simulink model "Carousel_SImulator"  (R2025a)
settings: Solver=VariableStepAuto  StartTime=0.0  StopTime=10.0  RelTol=1e-3
values from neighbouring files (symbols this model uses):
  initial_guess = homeConfiguration(robot)    [ik_solver_setup.m]
undefined symbols (not defined in the file or in its folder): exprnd, m, n, System
settings Model: Creator=samadhan  LastModifiedBy=samadhan

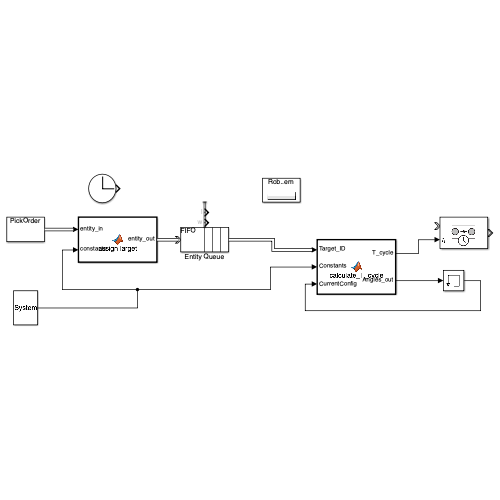
[thumbnail: Simulink's stored preview of the top-level diagram]
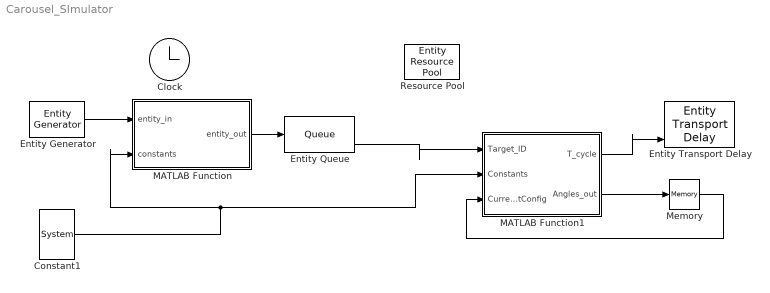
== system Carousel_SImulator ==
  Clock : Clock
  Constant1 : Constant  Value=System
  Entity Transport Delay : EntityTransportDelay  InputPortMessageModes=m,n  OutputPortMessageModes=m
  Entity Generator : EntityGenerator  OutputPortMessageModes=m  Period=eval('exprnd(10)')  IntergenerationTimeAction=exprnd(10)  AttributeName=Target_Bin_ID  EntityType=Structured  EntityTypeName=PickOrder  EntityPriority=1
  Entity Queue : Queue  InputPortMessageModes=m  OutputPortMessageModes=n,n,m  Capacity=inf  AverageWait=on  AverageQueueLength=on
      settings: OutputPortMap=o2,o3,o5
  MATLAB Function : MATLAB Function  TreatAsAtomicUnit=on
  MATLAB Function1 : MATLAB Function  TreatAsAtomicUnit=on
  Memory : Memory  InitialCondition=initial_guess
  Resource Pool : EntityResourcePool  ResourceName=RobotArmSystem  ResourceAmount=1
  wires:
  Constant1/1 -> MATLAB Function1/2(Constants), MATLAB Function/2(constants)
  MATLAB Function/1(entity_out) -> Entity Queue/1
  Entity Queue/3 -> MATLAB Function1/1(Target_ID)
  MATLAB Function1/1(T_cycle) -> Entity Transport Delay/2
  MATLAB Function1/2(Angles_out) -> Memory/1
  Memory/1 -> MATLAB Function1/3(CurrentConfig)
  Entity Generator/1 -> MATLAB Function/1(entity_in)

== matlab function Carousel_SImulator/MATLAB Function1 ==
  data: Target_ID input; T_cycle output; Constants input; CurrentConfig input; Angles_out output
function [T_cycle, Angles_out] = calculate_T_cycle(Target_ID, Constants, CurrentConfig)

    % Use coder.extrinsic to tell Simulink to execute these functions in MATLAB.
    coder.extrinsic('homeConfiguration', 'get_bin_position', ...
                    'calculate_retrieval_time', 'trvec2tform', 'step', 'evalin');
    
    % --- Load Workspace Objects ---
    % Since IK/Robot objects cannot be passed easily via signal lines, 
    % we must load them from the base workspace using evalin.
    % Note: These must exist in the base workspace (run your setup scripts first!).
    Robot = evalin('base', 'robot');
    IK = evalin('base', 'ik');
    Weights = evalin('base', 'weights');
    
    % --- A. Calculate Carousel Rotation Time (T_rot) ---
    [~, T_rot, T_grab_fixed] = calculate_retrieval_time(1, Target_ID, Constants);
    
    % --- B. Determine Grabber Target and Solve IK ---
    
    % 1. Get Target XYZ (position when the bin is at the access port)
    target_xyz = get_bin_position(1, Constants); 

    % 2. Define Target Pose (Position + Orientation)
    % Example orientation: The gripper needs to approach the bin.
    R_orientation = [0 0 1; 1 0 0; 0 1 0]; % Needs customization based on your arm's configuration
    T_target = [R_orientation, target_xyz'; 0 0 0 1];
    
    % 3. Solve IK: Calculate the target joint angles (angles_target)
    [angles_target, solution_info] = step(IK, T_target, Weights, CurrentConfig);

    % --- C. Dynamic T_grab Calculation ---
    
    % 1. Calculate the required joint movement (radians)
    Delta_Theta = abs(angles_target - CurrentConfig);
    
    % 2. Define Robot Joint Velocity Limits (Example: Should be in your constants)
    % Assuming a max joint velocity of 1.0 rad/s
    Max_Joint_Velocity = 1.0; 

    % 3. Time required for motion is determined by the joint that moves the most
    T_motion = max(Delta_Theta / Max_Joint_Velocity);
    
    % T_grab = Time to move + Fixed time for actuation/retraction (e.g., 1.5 seconds)
    T_grab_dynamic = T_motion + 1.5; 

    % --- D. Final Output ---
    T_cycle = T_rot + T_grab_dynamic;
    Angles_out = angles_target; % New state for the Memory block
end

== matlab function Carousel_SImulator/MATLAB Function ==
  data: entity_in input; entity_out output; constants input
function entity_out = assignTarget(entity_in, constants)
% ASSIGNTARGET Assigns a random bin ID to the PickOrder entity.

    % Get the total number of columns from the input constants structure
    N_cols = constants.System.N_Columns;

    % Generate a random integer between 1 and N_cols (inclusive)
    % This defines the location of the parcel that needs to be retrieved
    target_bin = randi([1, N_cols]); 

    % Write the generated random value to the entity's attribute
    entity_in.Target_Bin_ID = target_bin;

    % Output the modified entity
    entity_out = entity_in;
end
